simulink model "Simulink_7"  (Simulink 10.0)
settings: Solver=ode45  StartTime=0.0  StopTime=50.0  RelTol=1e-6  AbsTol=1e-6  EnableMultiTasking=on
libraries: simulink x1
settings Model: Creator=unknown  LastModifiedBy=unknown
settings DataIOCC: LimitDataPoints=on  SignalLoggingSaveFormat=ModelDataLogs  SignalLoggingName=sigsOut
settings OptimizationCC: LifeSpan=auto
settings DebuggingCC: SaveWithParameterizedLinksMsg=none  SignalResolutionControl=TryResolveAllWithWarning  MultiTaskDSMMsg=warning  MultiTaskCondExecSysMsg=none  SFUnexpectedBacktrackingDiag=error  SFNoUnconditionalDefaultTransitionDiag=error  SFExecutionAtInitializationDiag=warning  ArithmeticOperatorsInVariantConditions=error
settings HardwareCC: TargetUnknown=on
settings SFSimCC: SimUseLocalCustomCode=on  CustomCodeUndefinedFunction=FilterOut
settings RTWCC: RTWUseLocalCustomCode=on
settings CodeAppCC: StateflowObjectComments=off
settings GRTTargetCC: TargetLangStandard=C99 (ISO)

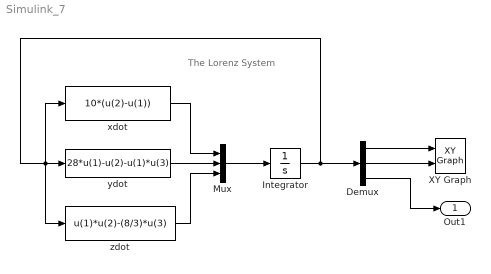
== system Simulink_7 ==
  note: The Lorenz System
  Demux : Demux  Outputs=3
  Integrator : Integrator  InitialCondition=[15 20 30]  UpperSaturationLimit=50  LowerSaturationLimit=0
  Mux : Mux  Inputs=3
  XY Graph : simulink/Sinks/XY Graph  xmin=-30  xmax=30  ymin=-30  ymax=30  st=-1
  xdot : Fcn  Description=sdhdkbkdf  Expr=10*(u(2)-u(1))
  ydot : Fcn  Expr=28*u(1)-u(2)-u(1)*u(3)
  zdot : Fcn  Expr=u(1)*u(2)-(8/3)*u(3)
  Out1 : Outport
  wires:
  xdot/1 -> Mux/1
  ydot/1 -> Mux/2
  zdot/1 -> Mux/3
  Mux/1 -> Integrator/1
  Integrator/1 -> ydot/1, xdot/1, zdot/1, Demux/1
  Demux/1 -> XY Graph/1
  Demux/2 -> XY Graph/2
  Demux/3 -> Out1/1
